simulink model "NCarState"  (R2024b)
settings: configuration reference "STM32H7_Config" (kept outside this file)
settings Model: DataDictionary=Master_Dictionary.sldd  EnableAccessToBaseWorkspace=off  Creator=torni  LastModifiedBy=William
settings ConfigSetRef: SourceName=STM32H7_Config

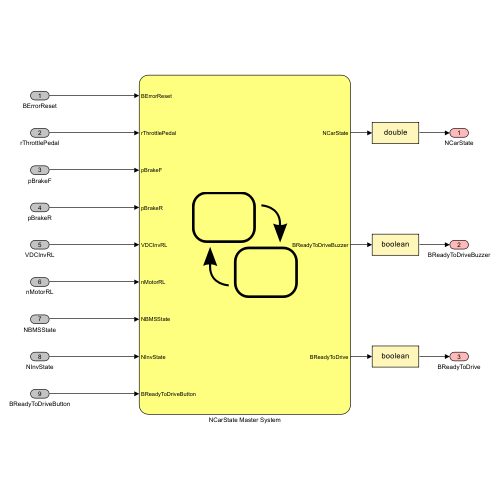
[thumbnail: Simulink's stored preview of the top-level diagram]
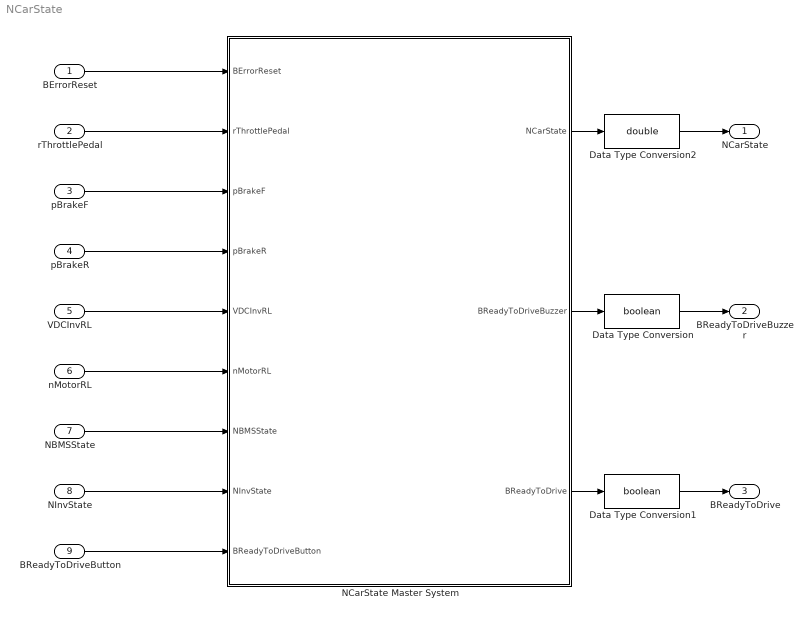
== system NCarState ==
  "BErrorReset " : Inport  OutDataTypeStr=boolean
  "rThrottlePedal " : Inport  Port=2  OutDataTypeStr=double
  "pBrakeF " : Inport  Port=3  OutDataTypeStr=double
  "pBrakeR " : Inport  Port=4  OutDataTypeStr=double
  VDCInvRL : Inport  Port=5  OutDataTypeStr=double
  "nMotorRL " : Inport  Port=6  OutDataTypeStr=double
  NBMSState : Inport  Port=7  OutDataTypeStr=double
  NInvState : Inport  Port=8  OutDataTypeStr=double
  BReadyToDriveButton : Inport  Port=9  OutDataTypeStr=boolean
  Data Type Conversion : DataTypeConversion  OutDataTypeStr=boolean  SaturateOnIntegerOverflow=off  RndMeth=Floor
  Data Type Conversion1 : DataTypeConversion  OutDataTypeStr=boolean  SaturateOnIntegerOverflow=off  RndMeth=Floor
  Data Type Conversion2 : DataTypeConversion  OutDataTypeStr=double  SaturateOnIntegerOverflow=off  RndMeth=Floor
  NCarState Master System : Stateflow chart  TreatAsAtomicUnit=on
  NCarState : Outport  OutDataTypeStr=double  VectorParamsAs1DForOutWhenUnconnected=off
  BReadyToDriveBuzzer : Outport  Port=2  OutDataTypeStr=boolean  VectorParamsAs1DForOutWhenUnconnected=off
  BReadyToDrive : Outport  Port=3  OutDataTypeStr=boolean  VectorParamsAs1DForOutWhenUnconnected=off
  wires:
  "nMotorRL "/1 -> NCarState Master System/6(nMotorRL)
  "BErrorReset "/1 -> NCarState Master System/1(BErrorReset)
  "rThrottlePedal "/1 -> NCarState Master System/2(rThrottlePedal)
  "pBrakeR "/1 -> NCarState Master System/4(pBrakeR)
  VDCInvRL/1 -> NCarState Master System/5(VDCInvRL)
  "pBrakeF "/1 -> NCarState Master System/3(pBrakeF)
  NBMSState/1 -> NCarState Master System/7(NBMSState)
  NInvState/1 -> NCarState Master System/8(NInvState)
  NCarState Master System/1(NCarState) -> Data Type Conversion2/1
  NCarState Master System/2(BReadyToDriveBuzzer) -> Data Type Conversion/1
  NCarState Master System/3(BReadyToDrive) -> Data Type Conversion1/1
  Data Type Conversion/1 -> BReadyToDriveBuzzer/1
  Data Type Conversion1/1 -> BReadyToDrive/1
  BReadyToDriveButton/1 -> NCarState Master System/9(BReadyToDriveButton)
  Data Type Conversion2/1 -> NCarState/1

== stateflow chart NCarState/NCarState Master System ==
  state Car_ON
    entry:
    NCarState=92;
    state ON
      entry:
      BReadyToDrive=1;
    (default) -> ON
  state Car_Idle_1
    entry:
    NCarState=0
  state Status_Check1
    entry:
    NCarState=1;
  note: here is where bmsstate==92 goes
  state BMS_Status_OK
    entry:
    NCarState=2;
  state Ready_To_Drive
    state RTD1
      entry:
      NCarState=6
      BReadyToDriveBuzzer=0
    state RTD_Sound
      entry:
      NCarState=5
      BReadyToDriveBuzzer=1
    RTD_Sound -> RTD1 : after(1500,tick)
    (default) -> RTD_Sound
  state Inv_LV_OK
    entry:
    NCarState=3;
  state Inv_HV_OK
    entry:
    NCarState=4;
  (default) -> Car_Idle_1
  Car_Idle_1 -> Status_Check1 : after(7000, tick)
  Car_ON -> Status_Check1 : [VDCInvRL<60]
  Inv_HV_OK -> Status_Check1 [order 1] : [(BErrorReset==1 &&...
      | nMotorRL<500) ||...
      | (VDCInvRL<60)]
  Ready_To_Drive -> Status_Check1 : [VDCInvRL<60]
  Status_Check1 -> BMS_Status_OK : after(500,tick)
  RTD1 -> Car_ON : [rThrottlePedal<=5]
  BMS_Status_OK -> Inv_LV_OK : [NInvState == 3]
  Inv_LV_OK -> Inv_HV_OK : [NInvState == 92]
  Inv_HV_OK -> Ready_To_Drive [order 2] : [NInvState == 92 &&...
      | rThrottlePedal<=5 &&...
      | BReadyToDriveButton==1 &&...
      | pBrakeF >= 3 &&...
      | pBrakeR >= 3]
  data: BErrorReset input boolean; NCarState output double; rThrottlePedal input double; pBrakeF input double; pBrakeR input double; VDCInvRL input double; nMotorRL input double; BReadyToDriveBuzzer output double; BReadyToDrive output double; NBMSState input double; NInvState input double; BReadyToDriveButton input boolean
